simulink library "navlib2"  (Simulink 2.09)
undefined symbols (not defined in the file or in its folder): HVOR, xVOR, yVOR
libraries: navlib2 x2

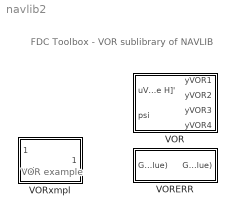
== system navlib2 ==
  note: FDC Toolbox - VOR sublibrary of NAVLIB
  note: VOR example
  VOR : Subsystem  mask(VOR){xVOR=xVOR, yVOR=yVOR, HVOR=HVOR}
      mask prompts: xVOR "x-position VOR relative to aircraft at t=0 sec. [m]:"; yVOR "y-position VOR relative to aircraft at t=0 sec. [m]:"; HVOR "Altitude of VOR in [m] above sea level:"
      mask help:
      | Calculation of nominal
      | VOR signals
      mask init:
      | CD=@4*pi/180;
      mask Help: eval('fdchelp vor')
      mask Display: disp('Nominal\nVOR\nsignals')
  VORERR : Subsystem  mask(VOR error){@1=5}
      mask prompts: @1 "Overall VOR system error [%]:"
      mask help: Steady-state error VOR
      mask init:
      | KVORerr = 1 + (@1/100);
      mask Help: eval('fdchelp vorerr')
      mask Display: disp('VOR Steady-\nstate error')
  VORxmpl : Subsystem
      mask Display: plot(0,0,100,100,[86,85,90,86,80,85,0],[16,80,20,16,20,80,62],[22,18,25,28,22,19],[36,32,29,33,36,45],[17,15,12,18,16,19],[37,37,34,32,44,46],[22,31,47,52,19,15,28,22],[36,44,39,44,55,50,45,38],[31,28],[44,45],[20,18,17],[31,30,32],[36,35,36,37,36,35,35,35,33,31,25],[41,38,33,32,30,30,32,33,37,35,34],[85,42],[80,50],[86,87,87,86,84,83,84,85],[83,81,78,76,76,79,82,83])

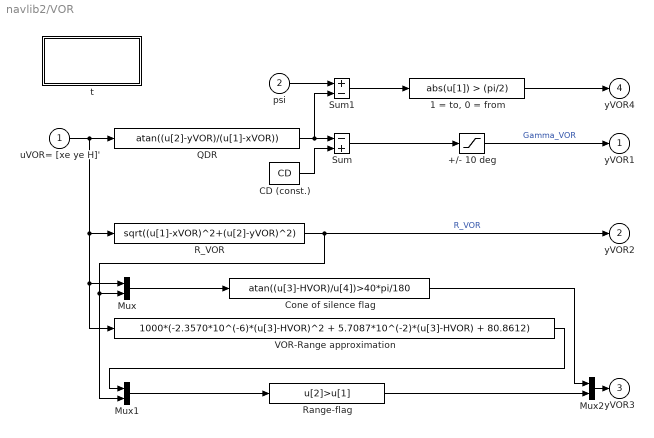
== system navlib2/VOR ==
  uVOR= [xe ye H]' : Inport  Port=1  PortWidth=-1  SampleTime=-1
  psi : Inport  Port=2  PortWidth=-1  SampleTime=-1
  +/- 10 deg : Saturate  UpperLimit=10*pi/180  LowerLimit=-10*pi/180
  "1 = to, 0 = from" : Fcn  Expr=abs(u[1]) > (pi/2)
  CD (const.) : Constant  Value=CD
  Cone of silence flag : Fcn  Expr=atan((u[3]-HVOR)/u[4])>40*pi/180
  Mux : Mux  Inputs=[3 1]
  Mux1 : Mux  Inputs=2
  Mux2 : Mux  Inputs=2
  QDR : Fcn  Expr=atan((u[2]-yVOR)/(u[1]-xVOR))
  R_VOR : Fcn  Expr=sqrt((u[1]-xVOR)^2+(u[2]-yVOR)^2)
  Range-flag : Fcn  Expr=u[2]>u[1]
  Sum : Sum  Inputs=-+
  Sum1 : Sum  Inputs=+-
  VOR-Range approximation : Fcn  Expr=1000*(-2.3570*10^(-6)*(u[3]-HVOR)^2 + 5.7087*10^(-2)*(u[3]-HVOR) + 80.8612)
  t : Subsystem
      settings: OpenFcn=fdchelp vor
      mask Display: disp('VOR signals\nMarc Rauw\nOctober 1997')
  yVOR1 : Outport  Port=1  InitialOutput=0
  yVOR2 : Outport  Port=2  InitialOutput=0
  yVOR3 : Outport  Port=3  InitialOutput=0
  yVOR4 : Outport  Port=4  InitialOutput=0
  wires:
  uVOR= [xe ye H]'/1 -> QDR/1, R_VOR/1, Mux/1, VOR-Range approximation/1
  "1 = to, 0 = from"/1 -> yVOR4/1
  CD (const.)/1 -> Sum/2
  Mux/1 -> Cone of silence flag/1
  R_VOR/1 -> yVOR2/1, Mux/2, Mux1/2  "R_VOR"
  Mux1/1 -> Range-flag/1
  Range-flag/1 -> Mux2/2
  VOR-Range approximation/1 -> Mux1/1
  Mux2/1 -> yVOR3/1
  QDR/1 -> Sum/1, Sum1/2
  psi/1 -> Sum1/1
  Sum1/1 -> "1 = to, 0 = from"/1
  +/- 10 deg/1 -> yVOR1/1  "Gamma_VOR"
  Sum/1 -> +/- 10 deg/1
  Cone of silence flag/1 -> Mux2/1

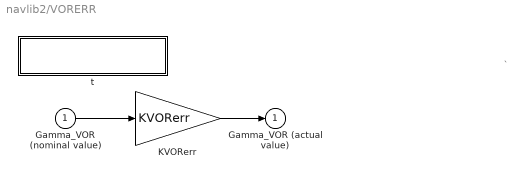
== system navlib2/VORERR ==
  note: `
  Gamma_VOR (nominal value) : Inport  Port=1  PortWidth=-1  SampleTime=-1
  KVORerr : Gain  Gain=KVORerr
  t : Subsystem
      settings: OpenFcn=fdchelp vorerr
      mask Display: disp('VOR steady-state error\nMarc Rauw, October 1997')
  Gamma_VOR (actual value) : Outport  Port=1  InitialOutput=0
  wires:
  Gamma_VOR (nominal value)/1 -> KVORerr/1
  KVORerr/1 -> Gamma_VOR (actual value)/1

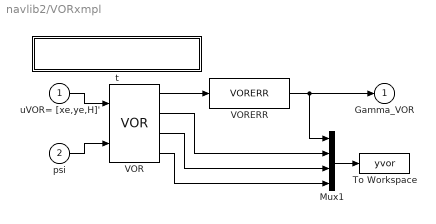
== system navlib2/VORxmpl ==
  uVOR= [xe,ye,H]' : Inport  Port=1  PortWidth=-1  SampleTime=-1
  psi : Inport  Port=2  PortWidth=-1  SampleTime=-1
  Mux1 : Mux  Inputs=[1 1 2 1]
  To Workspace : ToWorkspace  VariableName=yvor  SampleTime=0
      settings: Buffer=5000
  VOR : navlib2/VOR  xVOR=xVOR  yVOR=yVOR  HVOR=HVOR  MaskParam4=CD
  VORERR : navlib2/VORERR  MaskParam1=5
  t : Subsystem
      settings: OpenFcn=fdchelp vorxmpl
      mask Display: disp('VOR example\nMarc Rauw, January 1998')
  Gamma_VOR : Outport  Port=1  InitialOutput=0
  wires:
  VOR/1 -> VORERR/1
  Mux1/1 -> To Workspace/1
  VOR/2 -> Mux1/2
  VOR/3 -> Mux1/3
  VOR/4 -> Mux1/4
  psi/1 -> VOR/2
  uVOR= [xe,ye,H]'/1 -> VOR/1
  VORERR/1 -> Gamma_VOR/1, Mux1/1

== system navlib2/VOR/t ==

== system navlib2/VORERR/t ==

== system navlib2/VORxmpl/t ==
